simulink model "flexible_drive_q34_collocated"  (Simulink 10.1)
settings: Solver=ode45  StartTime=0.0  StopTime=4  RelTol=1e-3  EnableMultiTasking=on
values from neighbouring files (symbols this model uses):
  b1 = b_1    [three_one.m]    (also in three_two.m = 0.01)
  b2 = b_2    [three_one.m]    (also in three_two.m = 0.001)
  c = 0    [three_one.m]    (also in three_two.m)
  d1 = d_1    [three_one.m]    (also in three_two.m = 0.846)
  d2 = d_2    [three_one.m]    (also in three_two.m = 0.0846)
  k = m_1 * m_2 * w_n^2 / m_t    [three_one.m]    (also in three_two.m = 0.0473)
  k_p = 0.19    [three_one.m]
  m1 = m_1    [three_one.m]    (also in three_two.m = 0.000321)
  m2 = m_2    [three_one.m]    (also in three_two.m = 0.000174)
  Ts = 0.001    [three_one.m]    (also in three_two.m)
undefined symbols (not defined in the file or in its folder): sgn
settings Model: Creator=user  LastModifiedBy=Kaelan
settings DataIOCC: LimitDataPoints=on  SignalLoggingSaveFormat=ModelDataLogs  SignalLoggingName=sigsOut
settings DebuggingCC: SaveWithParameterizedLinksMsg=none  SignalResolutionControl=TryResolveAllWithWarning  MultiTaskDSMMsg=warning  MultiTaskCondExecSysMsg=none  SFExecutionAtInitializationDiag=warning
settings HardwareCC: TargetUnknown=on
settings ConfigComp: CovHtmlReporting=off

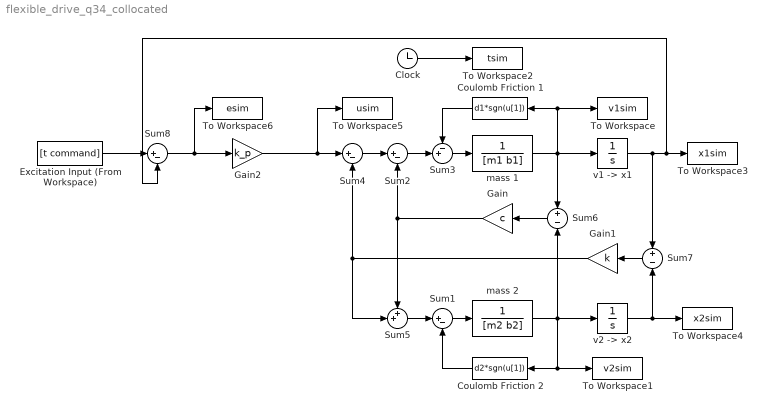
== system flexible_drive_q34_collocated ==
  Clock : Clock
  Coulomb Friction 1 : Fcn  Expr=d1*sgn(u[1])
  Coulomb Friction 2 : Fcn  Expr=d2*sgn(u[1])
  Excitation Input (From Workspace) : FromWorkspace  VariableName=[t command]  SampleTime=Ts  ZeroCross=off  OutputAfterFinalValue=Holding final value
  Gain : Gain  Gain=c  SaturateOnIntegerOverflow=on  OutDataTypeStr=Inherit: Same as input  ParamDataTypeStr=Inherit: Same as input
  Gain1 : Gain  Gain=k  SaturateOnIntegerOverflow=on  OutDataTypeStr=Inherit: Same as input  ParamDataTypeStr=Inherit: Same as input
  Gain2 : Gain  Gain=k_p
  Sum{1..2,4,8} (4 alike) : Sum  Inputs=|+-  SaturateOnIntegerOverflow=on
  Sum3 : Sum  Inputs=-+|  SaturateOnIntegerOverflow=on
  Sum5 : Sum  Inputs=++|  SaturateOnIntegerOverflow=on
  Sum6 : Sum  Inputs=+|-  SaturateOnIntegerOverflow=on
  Sum7 : Sum  Inputs=+|-  SaturateOnIntegerOverflow=on
  To Workspace : ToWorkspace  VariableName=v1sim  SampleTime=Ts
  To Workspace1 : ToWorkspace  VariableName=v2sim  SampleTime=Ts
  To Workspace2 : ToWorkspace  VariableName=tsim  SampleTime=Ts
  To Workspace3 : ToWorkspace  VariableName=x1sim  SampleTime=Ts
  To Workspace4 : ToWorkspace  VariableName=x2sim  SampleTime=Ts
  To Workspace5 : ToWorkspace  VariableName=usim  SampleTime=Ts
  To Workspace6 : ToWorkspace  VariableName=esim  SampleTime=Ts
  mass 1 : TransferFcn  Denominator=[m1 b1]
  mass 2 : TransferFcn  Denominator=[m2 b2]
  "v1 -> x1" : Integrator
  "v2 -> x2" : Integrator
  wires:
  mass 1/1 -> "v1 -> x1"/1, Sum6/1, Coulomb Friction 1/1, To Workspace/1
  Clock/1 -> To Workspace2/1
  Sum3/1 -> mass 1/1
  Coulomb Friction 1/1 -> Sum3/1
  mass 2/1 -> "v2 -> x2"/1, Sum6/2, Coulomb Friction 2/1, To Workspace1/1
  Sum1/1 -> mass 2/1
  Coulomb Friction 2/1 -> Sum1/2
  Sum2/1 -> Sum3/2
  Sum5/1 -> Sum1/1
  Sum6/1 -> Gain/1
  Gain/1 -> Sum2/2, Sum5/1
  "v1 -> x1"/1 -> Sum8/2, To Workspace3/1, Sum7/1
  "v2 -> x2"/1 -> Sum7/2, To Workspace4/1
  Sum7/1 -> Gain1/1
  Gain1/1 -> Sum4/2, Sum5/2
  Sum4/1 -> Sum2/1
  Excitation Input (From Workspace)/1 -> Sum8/1
  Gain2/1 -> Sum4/1, To Workspace5/1
  Sum8/1 -> To Workspace6/1, Gain2/1
